simulink model "L2_1"  (R2021b)
settings: Solver=ode4  StartTime=0.0  StopTime=50  FixedStep=0.001  RelTol=1e-3
settings Model: Creator=george.tudor1906  LastModifiedBy=george.tudor1906

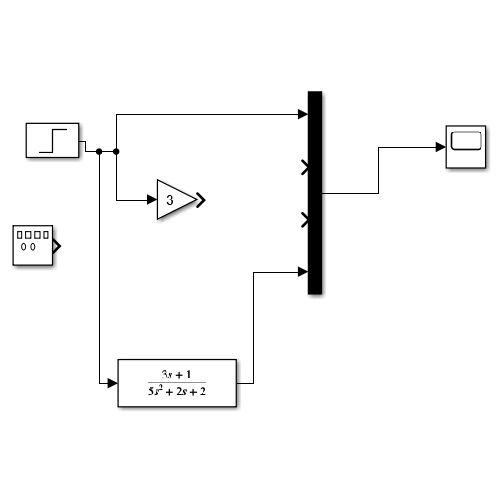
[thumbnail: Simulink's stored preview of the top-level diagram]
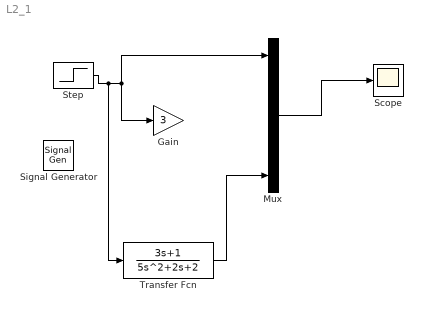
== system L2_1 ==
  Gain : Gain  Gain=3
  Mux : Mux
  Scope : Scope
  Signal Generator : SignalGenerator  Amplitude=10  Units=rad/sec
  Step : Step  Time=5  After=10  SampleTime=0
  Transfer Fcn : TransferFcn  Numerator=[3 1]  Denominator=[5 2 2]
  wires:
  Mux/1 -> Scope/1
  Step/1 -> Transfer Fcn/1, Mux/1, Gain/1
  Transfer Fcn/1 -> Mux/4
